simulink model "adaptive_dcmotor"  (R2025b)
settings: Solver=FixedStepAuto  StartTime=0.0  StopTime=inf  FixedStep=0.08  RelTol=1e-3  EnableMultiTasking=on
libraries: arduinolib x3, arduinosensorlib x1
settings Model: Creator=Lenard  LastModifiedBy=Lenard
settings SolverCC: AutoInsertRateTranBlk=on
settings OptimizationCC: EnhancedBackFolding=on  PassReuseOutputArgsAs=Individual arguments  ZeroExternalMemoryAtStartup=off  ZeroInternalMemoryAtStartup=off  MaxStackSize=64  OptimizeBlockOrder=speed  DifferentSizesBufferReuse=on  OptimizationCustomize=off  EfficientTunableParamExpr=on
settings DebuggingCC: ParameterTunabilityLossMsg=error
settings HardwareCC: ProdBitPerPointer=32.0  ProdBitPerSizeT=32.0  ProdBitPerPtrDiffT=32.0  ProdLargestAtomicInteger=Long  ProdLargestAtomicFloat=Double  ProdWordSize=32.0  ProdHWDeviceType=ARM Compatible->ARM Cortex
settings SFSimCC: MATLABDynamicMemAlloc=off
settings RTWCC: SystemTargetFile=ert.tlc  HardwareBoard=ESP32-WROOM (Arduino Compatible)  TLCOptions="-aInlineSetEventsForThisBaseRateFcn=TLC_FALSE -aSuppressMultiTaskScheduler=TLC_FALSE  -aRateBasedStepFcn=0"  TemplateMakefile=ert_default_tmf  Toolchain=ESP32  BuildConfiguration=Faster Runs  Description=Embedded Coder
settings CodeAppCC: ForceParamTrailComments=on  IgnoreCustomStorageClasses=off  OperatorAnnotations=on  SimulinkDataObjDesc=on  SFDataObjDesc=on  InsertBlockDesc=on
settings ERTTargetCC: ExtModeTransport=3.0  ExtModeStaticAlloc=on  ExtModeAutomaticAllocSize=off  ExtModeStaticAllocSize=65536.0  ExtModeMexFile=ext_xcp  ExtModeIntrfLevel=Level2 - Open  InlinedParameterPlacement=Hierarchical  SupportContinuousTime=on  SupportVariableSizeSignals=on

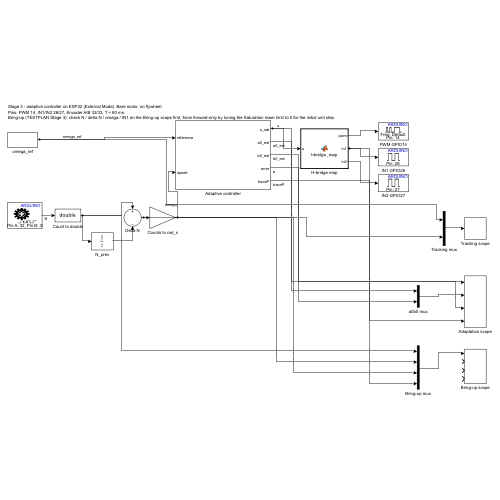
[thumbnail: Simulink's stored preview of the top-level diagram]
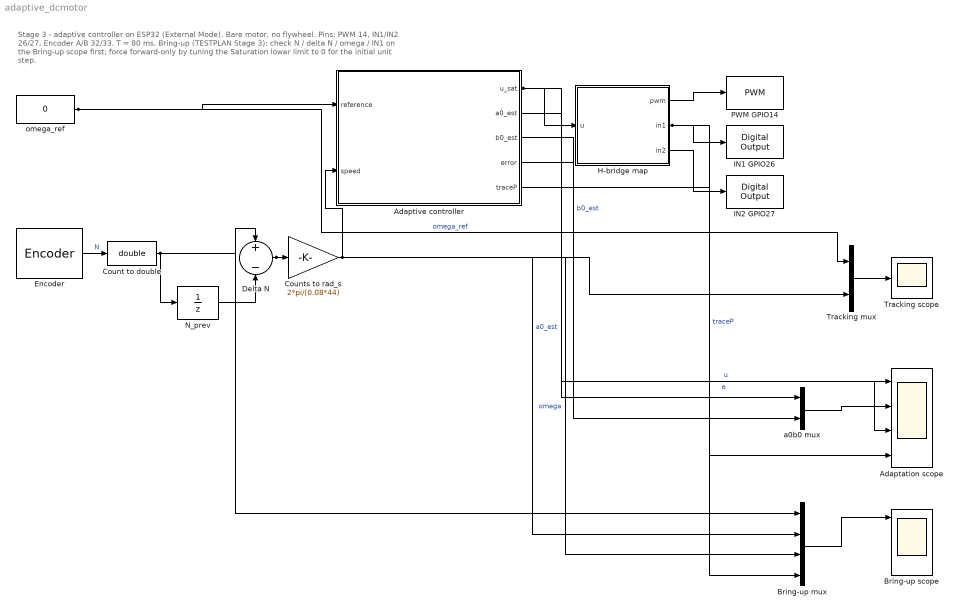
== system adaptive_dcmotor ==
  note: Stage 3 - adaptive controller on ESP32 (External Mode). Bare motor, no flywheel.
      | Pins: PWM 14, IN1/IN2 26/27, Encoder A/B 32/33. T = 80 ms.
      | Bring-up (TESTPLAN Stage 3): check N / delta N / omega / IN1 on the Bring-up scope first; force forward-only by tuning the Saturation lower limit to 0 for the initial unit step.
  Adaptation scope : Scope  NumInputPorts=4
  Adaptive controller : Subsystem
  Bring-up mux : Mux
  Bring-up scope : Scope  NumInputPorts=4
  Count to double : DataTypeConversion  OutDataTypeStr=double  SaturateOnIntegerOverflow=off  RndMeth=Floor
  Counts to rad_s : Gain  Gain=2*pi/(0.08*44)
  Delta N : Sum  Inputs=+-
  Encoder : arduinosensorlib/Encoder  InputA=32  InputB=33  Mode=No reset  SampleTime=0.08
  H-bridge map : MATLAB Function  TreatAsAtomicUnit=on
  IN1 GPIO26 : arduinolib/Digital Output  pinNumber=26  Direction=output  blockPlatform=arduino
  IN2 GPIO27 : arduinolib/Digital Output  pinNumber=27  Direction=output  blockPlatform=arduino
  N_prev : UnitDelay  SampleTime=0.08  HasFrameUpgradeWarning=on
  PWM GPIO14 : arduinolib/PWM  pinNumber=14  frequencyType=Default  desiredFrequency=490.2  achievableFrequency=490.2
  Tracking mux : Mux  Inputs=2
  Tracking scope : Scope
  a0b0 mux : Mux  Inputs=2
  omega_ref : Constant  Value=0  SampleTime=0.08
  wires:
  omega_ref/1 -> Adaptive controller/1(reference), Tracking mux/1  "omega_ref"
  Encoder/1 -> Count to double/1  "N"
  Count to double/1 -> Delta N/1, N_prev/1, Bring-up mux/1
  N_prev/1 -> Delta N/2
  Delta N/1 -> Counts to rad_s/1, Bring-up mux/2
  Counts to rad_s/1 -> Adaptive controller/2(speed), Tracking mux/2, Bring-up mux/3  "omega"
  Adaptive controller/1(u_sat) -> H-bridge map/1(u), Adaptation scope/1  "u"
  H-bridge map/1(pwm) -> PWM GPIO14/1
  H-bridge map/2(in1) -> IN1 GPIO26/1, Bring-up mux/4
  H-bridge map/3(in2) -> IN2 GPIO27/1
  Tracking mux/1 -> Tracking scope/1
  Adaptive controller/2(a0_est) -> a0b0 mux/1  "a0_est"
  Adaptive controller/3(b0_est) -> a0b0 mux/2  "b0_est"
  a0b0 mux/1 -> Adaptation scope/2
  Adaptive controller/4(error) -> Adaptation scope/3  "e"
  Adaptive controller/5(traceP) -> Adaptation scope/4  "traceP"
  Bring-up mux/1 -> Bring-up scope/1

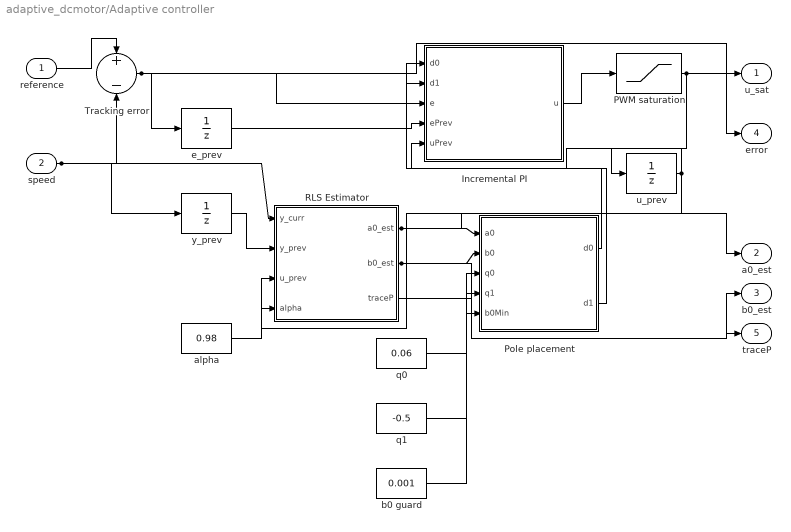
== system adaptive_dcmotor/Adaptive controller ==
  reference : Inport
  speed : Inport  Port=2
  Incremental PI : MATLAB Function  TreatAsAtomicUnit=on
  PWM saturation : Saturate  UpperLimit=255  LowerLimit=-255
  Pole placement : MATLAB Function  TreatAsAtomicUnit=on
  RLS Estimator : MATLAB Function  TreatAsAtomicUnit=on
  Tracking error : Sum  Inputs=+-
  alpha : Constant  Value=0.98
  b0 guard : Constant  Value=0.001
  e_prev : UnitDelay  SampleTime=0.08  HasFrameUpgradeWarning=on
  q0 : Constant  Value=0.06
  q1 : Constant  Value=-0.5
  u_prev : UnitDelay  SampleTime=0.08  HasFrameUpgradeWarning=on
  y_prev : UnitDelay  SampleTime=0.08  HasFrameUpgradeWarning=on
  u_sat : Outport
  a0_est : Outport  Port=2
  b0_est : Outport  Port=3
  error : Outport  Port=4
  traceP : Outport  Port=5
  wires:
  reference/1 -> Tracking error/1
  speed/1 -> Tracking error/2, y_prev/1, RLS Estimator/1(y_curr)
  Tracking error/1 -> e_prev/1, Incremental PI/3(e), error/1
  y_prev/1 -> RLS Estimator/2(y_prev)
  u_prev/1 -> RLS Estimator/3(u_prev), Incremental PI/5(uPrev)
  alpha/1 -> RLS Estimator/4(alpha)
  RLS Estimator/1(a0_est) -> Pole placement/1(a0), a0_est/1
  RLS Estimator/2(b0_est) -> Pole placement/2(b0), b0_est/1
  RLS Estimator/3(traceP) -> traceP/1
  q0/1 -> Pole placement/3(q0)
  q1/1 -> Pole placement/4(q1)
  b0 guard/1 -> Pole placement/5(b0Min)
  Pole placement/1(d0) -> Incremental PI/1(d0)
  Pole placement/2(d1) -> Incremental PI/2(d1)
  e_prev/1 -> Incremental PI/4(ePrev)
  Incremental PI/1(u) -> PWM saturation/1
  PWM saturation/1 -> u_prev/1, u_sat/1

== matlab function adaptive_dcmotor/Adaptive controller/Pole placement ==
  data: a0 input; d0 output; b0 input; q0 input; q1 input; b0Min input; d1 output
function [d0,d1] = pole_placement(a0,b0,q0,q1,b0Min)            
                                                               %#codegen                                                       
                                                               % Hold the previous gains while |b0| is too small (guard against
                                                               % division blow-up before the estimator has converged).         
                                                               persistent d0Hold d1Hold                                        
                                                               if isempty(d0Hold)                                              
                                                                   d0Hold = -0.44;                                             
                                                                   d1Hold = 1.0;                                               
                                                               end                                                             
                                                               if abs(b0) > b0Min                                              
                                                                   d0Hold = (q0 + a0) / b0;                                    
                                                                   d1Hold = (q1 + 1.0 - a0) / b0;                              
                                                               end                                                             
                                                               d0 = d0Hold;                                                    
                                                               d1 = d1Hold;                                                    
                                                               end

== matlab function adaptive_dcmotor/Adaptive controller/RLS Estimator ==
  data: y_curr input; a0_est output; y_prev input; u_prev input; alpha input; b0_est output; traceP output
function [a0_est,b0_est,traceP] = rls_estimator(y_curr,y_prev,u_prev,alpha)
                                                                          %#codegen                                                                  
                                                                          % RLS for G(z) = b0/(z + a0). Excitation gate: skip the update when        
                                                                          % the regressor is ~zero (motor idle) so P = P/alpha cannot wind up.       
                                                                          persistent P xe                                                            
                                                                          if isempty(P)                                                              
                                                                              P = 100.0 * eye(2);                                                    
                                                                              xe = [-0.5; 1.0];                                                      
                                                                          end                                                                        
                                                                          C = [-y_prev, u_prev];                                                     
                                                                          if (C * C') > 1e-6                                                         
                                                                              den = C * P * C' + alpha;                                              
                                                                              L = (P * C') / den;                                                    
                                                                              xe = xe + L * (y_curr - C * xe);                                       
                                                                              P = (eye(2) - L * C) * P / alpha;                                      
                                                                              P = 0.5 * (P + P');                                                    
                                                                          end                                                                        
                                                                          a0_est = xe(1);                                                            
                                                                          b0_est = xe(2);                                                            
                                                                          traceP = P(1,1) + P(2,2);                                                  
                                                                          end

== matlab function adaptive_dcmotor/Adaptive controller/Incremental PI ==
  data: d0 input; u output; d1 input; e input; ePrev input; uPrev input
function u = incremental_pi(d0,d1,e,ePrev,uPrev)
                                               %#codegen                                       
                                               u = uPrev + d1 * e + d0 * ePrev;                
                                               end

== matlab function adaptive_dcmotor/H-bridge map ==
  data: u input; pwm output; in1 output; in2 output
function [pwm,in1,in2] = hbridge_map(u)                    
                                                          %#codegen                                                  
                                                          % |u| -> PWM duty (0..255), sign(u) -> L298N direction pins
                                                          pwm = abs(u);                                              
                                                          if u >= 0                                                  
                                                              in1 = 1; in2 = 0;                                      
                                                          else                                                       
                                                              in1 = 0; in2 = 1;                                      
                                                          end                                                        
                                                          end
